simulink library "DQN_Lib"  (R2023b)
settings: Solver=VariableStepAuto  StartTime=0.0  StopTime=10.0  RelTol=1e-3
undefined symbols (not defined in the file): ACDC3, HRM, La, N, R, Ra, sps_AC, SYS, Ts, Ts_dqn, Ts_Power, w, Ws
libraries: DQN_Lib_bak x7
(part 3 of 3)

== matlab function DQN_Lib/Int_DQN/Int_d_2N_2 ==
  settings: updateMethod=DISCRETE
  data: Zdp output; Xdp input; Xdn input; Xdz input; Xqp input; Xqn input; Xqz input; Zdn output; N parameter; dt parameter; w parameter; EMT parameter; Zdz output; Zqp output; Zqn output; Zqz output; InitInt parameter; chkHrmLst parameter; HrmLst parameter
function [Zdp,Zdn,Zdz,Zqp,Zqn,Zqz]  = IntDQN(Xdp, Xdn, Xdz, Xqp, Xqn, Xqz, N, dt, w, EMT, InitInt, chkHrmLst, HrmLst)

    persistent Zdc_old;    
    persistent Xdc_old;   
    persistent Zdp_old;    
    persistent Zqp_old;    
    persistent Zdn_old;    
    persistent Zqn_old;    
    persistent Zdz_old;    
    persistent Zqz_old;  
       
    persistent HrmLst2;
    persistent dt2;
    persistent range;
    
    Xdc = zeros(6,1);
    Zdc = zeros(6,1);
    
    Xdc(1) = Xdp(1);
    Xdc(2) = Xdn(1);
    Xdc(3) = Xdz(1);
    Xdc(4) = Xqp(1);
    Xdc(5) = Xqn(1);
    Xdc(6) = Xqz(1);

    Xdp = [Xdp(2:end); zeros(N-numel(Xdp)+1,1)];
    Xqp = [Xqp(2:end); zeros(N-numel(Xqp)+1,1)];
    Xdn = [Xdn(2:end); zeros(N-numel(Xdn)+1,1)];
    Xqn = [Xqn(2:end); zeros(N-numel(Xqn)+1,1)];
    Xdz = [Xdz(2:end); zeros(N-numel(Xdz)+1,1)];
    Xqz = [Xqz(2:end); zeros(N-numel(Xqz)+1,1)];
       
    Zdp = zeros(N+1,1);
    Zdn = zeros(N+1,1);
    Zqp = zeros(N+1,1);
    Zqn = zeros(N+1,1);
    Zdz = zeros(N+1,1);
    Zqz = zeros(N+1,1);
    
    if(isempty(Zdc_old)) 
        Zdc_old  = InitInt';
        Xdc_old  = zeros(6,1);
        
        Zdp_old  = zeros(N,1); Zdp_old(1) = InitInt(1);
        Zdn_old  = zeros(N,1); Zdn_old(1) = InitInt(2);
        Zdz_old  = zeros(N,1); Zdz_old(1) = InitInt(3);
        Zqp_old  = zeros(N,1); Zqp_old(1) = InitInt(4);
        Zqn_old  = zeros(N,1); Zqn_old(1) = InitInt(5);
        Zqz_old  = zeros(N,1); Zqz_old(1) = InitInt(6);
        
        if(isempty(HrmLst2))            
            HrmLst2 = HrmLst;
            HrmLst2(HrmLst2==0) = [];
        end
        dt2 = dt/2;  
        
        if(chkHrmLst)
            range = numel(HrmLst2);
        else
            range = N; 
        end
        
    end

    
    
    Zdc(:) = dt2*(Xdc(:)+Xdc_old(:))+Zdc_old(:);
    Zdc_old = Zdc;
    Xdc_old = Xdc;


    if(N>0)
        A = 0;
        

        
        i = 1;

        for g = 1 : range
            
            if(chkHrmLst)
                if(HrmLst2(g)>0)
                    i = HrmLst2(g);
                end
            else
                i = g; 
            end
            
            
            wn =  i * w; 

            if(EMT)

                A = 2/(1+(dt2*wn)^2);
                %A = 1/(1+(dt2*wn)^2);

                wndt2 = wn*dt2;

                %%% POS %%%
                K1 = dt2*(2*Xdp(i)+Zqp_old(i)*wn) + Zdp_old(i);
                K2 = dt2*(2*Xqp(i)-Zdp_old(i)*wn) + Zqp_old(i);

                Zdp(i) = A*( K1 + wndt2*K2)/2;
                Zqp(i) = A*( K2 - wndt2*K1)/2;
                %Zdp(i) = A*( K1 + wndt2*K2);
                %Zqp(i) = A*( K2 - wndt2*K1);

                Zdp_old(i) = Zdp(i);
                Zqp_old(i) = Zqp(i); 

                %%% NEG %%%
                K1 = dt2*(2*Xdn(i)-Zqn_old(i)*wn) + Zdn_old(i);
                K2 = dt2*(2*Xqn(i)+Zdn_old(i)*wn) + Zqn_old(i);

                Zdn(i) = A*( K1 - wndt2*K2)/2;
                Zqn(i) = A*( K2 + wndt2*K1)/2;
                %Zdn(i) = A*( K1 - wndt2*K2);
                %Zqn(i) = A*( K2 + wndt2*K1);

                Zdn_old(i) = Zdn(i);
                Zqn_old(i) = Zqn(i);

                %%% ZERO %%%
                K1 = dt2*(2*Xdz(i)+Zqz_old(i)*wn) + Zdz_old(i);
                K2 = dt2*(2*Xqz(i)-Zdz_old(i)*wn) + Zqz_old(i);

                Zdz(i) = A*( K1 + wndt2*K2)/2;
                Zqz(i) = A*( K2 - wndt2*K1)/2;
                %Zdz(i) = A*( K1 + wndt2*K2);
                %Zqz(i) = A*( K2 - wndt2*K1);

                Zdz_old(i) = Zdz(i);
                Zqz_old(i) = Zqz(i);

            else
    
                Tad_p2 = (2/3)*[sin(0) sin(0-2*pi/3) sin(0+2*pi/3);  
                               cos(0) cos(0-2*pi/3) cos(0+2*pi/3);];

                Tad_z2 = (1/3)*[sin(0) sin(0) sin(0);  
                               cos(0) cos(0) cos(0);];

                Ta_dqn = [Tad_p2(1,:); Tad_p2(1,:); Tad_z2(1,:); Tad_p2(2,:); Tad_p2(2,:); Tad_z2(2,:)];

                Zdp(i) = (Xqp(i))*(1/(wn));
                Zqp(i) = (Xdp(i))*(-1/(wn)); 

                Zdn(i) = (Xqn(i))*(-1/(wn));
                Zqn(i) = (Xdn(i))*(1/(wn)); 

                Zdz(i) = (Xqz(i))*(1/(wn));
                Zqz(i) = (Xdz(i))*(-1/(wn));
                

                sT = sin(2*pi/3);
                cT = cos(2*pi/3);
%                 Zdc([1,4, 3]) = Zdc([1,4, 3])-Tad_p*[Zqp(i);-sT*Zdp(i)+cT*Zqp(i);sT*Zdp(i)+cT*Zqp(i)];
%                 Zdc([1,4, 3]) = Zdc([1,4, 3])-Tad_p*[Zqn(i);-sT*Zdn(i)+cT*Zqn(i);sT*Zdn(i)+cT*Zqn(i)];
%                 Zdc([1,4, 3]) = Zdc([1,4, 3])-Tad_p*[Zqz(i); Zqz(i)             ;Zqz(i)];

                Zdc = Zdc-Ta_dqn*[Zqp(i);-sT*Zdp(i)+cT*Zqp(i);sT*Zdp(i)+cT*Zqp(i)];
                Zdc = Zdc-Ta_dqn*[Zqn(i);-sT*Zdn(i)+cT*Zqn(i);sT*Zdn(i)+cT*Zqn(i)];
                Zdc = Zdc-Ta_dqn*[Zqz(i); Zqz(i)             ;Zqz(i)];

            end
            

        end

        Zdp(2:end) = Zdp(1:end-1);
        Zdn(2:end) = Zdn(1:end-1);
        Zdz(2:end) = Zdz(1:end-1);
        Zqp(2:end) = Zqp(1:end-1);
        Zqn(2:end) = Zqn(1:end-1);
        Zqz(2:end) = Zqz(1:end-1);


    end
    
    Zdp(1)     = Zdc(1);
    Zdn(1)     = Zdc(2);
    Zdz(1)     = Zdc(3);
    Zqp(1)     = Zdc(4);
    Zqn(1)     = Zdc(5);
    Zqz(1)     = Zdc(6);
end

== matlab function DQN_Lib/MATLAB Function9 ==
  data: Xdcpnz_c input; Y_DQN output
function Y_DQN  = f012C2DQN(Xdcpnz_c)

    if(size(Xdcpnz_c,2) < 2)
        error('Wrong size!');
    end
    
    N = size(Xdcpnz_c,2)-1;
    Y_DQN = zeros(N+1,6);

    Y_DQN(1,4) =  2*real(Xdcpnz_c(1,1));
    Y_DQN(1,5) =  2*real(Xdcpnz_c(2,1));
    Y_DQN(1,6) =  real(Xdcpnz_c(3,1));

    Y_DQN(1,1) =  -2*imag(Xdcpnz_c(1,1));
    Y_DQN(1,2) =  2*imag(Xdcpnz_c(2,1));
    Y_DQN(1,3) =  imag(Xdcpnz_c(3,1));
    
    for i = 2 : N + 1
    
        Y_DQN(i,1) =  real(Xdcpnz_c(1,i));
        Y_DQN(i,2) = -real(Xdcpnz_c(2,i));
        Y_DQN(i,3) =  real(Xdcpnz_c(3,i));

        Y_DQN(i,4) =  imag(Xdcpnz_c(1,i));
        Y_DQN(i,5) =  imag(Xdcpnz_c(2,i));
        Y_DQN(i,6) =  imag(Xdcpnz_c(3,i));
    
    end


end

== matlab function DQN_Lib/DQN2abc/DQn->ABC19 ==
  data: Xdp input; Xdn input; Xdz input; Xqp input; Xqn input; Xqz input; th input; abc output; N parameter
%function abc = Mult(Z0,Zdp,Zqp,Zdn,Zqn,Zdz,Zqz,th, N)
function abc = dqn2abc(Xdp,Xdn,Xdz,Xqp,Xqn,Xqz,th,N)

    %Xdc = zeros(1,6);
    Xdc = zeros(6,1);

    persistent Tda_p2;
    persistent Tdqn_a;
    
    if(isempty(Tda_p2)) 
        Tda_p2 = [-0           1     1;
                 -sqrt(3/4)  -0.5   1;
                  sqrt(3/4)  -0.5   1;];
                Tdqn_a = zeros(3,6);
                Tdqn_a = [Tda_p2(:,1)  Tda_p2(:,1)  0*Tda_p2(:,3)  Tda_p2(:,2)  Tda_p2(:,2)  2*Tda_p2(:,3)]/2;
    end


    Xdc(1) = Xdp(1);
    Xdc(2) = Xdn(1);
    Xdc(3) = Xdz(1);
    Xdc(4) = Xqp(1);
    Xdc(5) = Xqn(1);
    Xdc(6) = Xqz(1);

    abc = Tdqn_a*Xdc;

    abc3p = [0;0;0];
    abc3n = [0;0;0];
    abc1p = [0;0;0];
 

    for i = 1 : N

        Tda_p = [sin(i*th)          cos(i*th);
                 sin(i*th-2*pi/3)   cos(i*th-2*pi/3);
                 sin(i*th+2*pi/3)   cos(i*th+2*pi/3)];
        Tda_n = [sin(-i*th)         cos(-i*th);
                 sin(-i*th-2*pi/3)  cos(-i*th-2*pi/3);
                 sin(-i*th+2*pi/3)  cos(-i*th+2*pi/3)];
        Tda_z = [sin(i*th)          cos(i*th);
                 sin(i*th-0*pi/3)   cos(i*th-0*pi/3);
                 sin(i*th+0*pi/3)   cos(i*th+0*pi/3)];

        abc3p = abc3p + Tda_p*[Xdp(i+1);Xqp(i+1)];
        abc3n = abc3n + Tda_n*[Xdn(i+1);Xqn(i+1)];
        abc1p = abc1p + Tda_z*[Xdz(i+1);Xqz(i+1)];  

    end

    abc = abc+abc3p+abc3n+abc1p;%+abc1n;

== matlab function DQN_Lib/Add_DQN/MATLAB Function1 ==
  data: Xdp input; Xdn input; Xdz input; Xqp input; Xqn input; Xqz input; Ydp input; Ydn input; Ydz input; Yqp input; Yqn input; Yqz input; Zdp output; Zdn output; Zdz output; Zqp output; Zqn output; Zqz output; N parameter; chkHrmLst parameter; HrmLst parameter
function [Zdp,Zdn,Zdz,Zqp,Zqn,Zqz]  = SumDQN(Xdp, Xdn, Xdz, Xqp, Xqn, Xqz, Ydp, Ydn, Ydz, Yqp, Yqn, Yqz, N, chkHrmLst, HrmLst)
%function [Zdc,Zdp,Zqp,Zdn,Zqn,Zdz,Zqz]  = SumDQN(Xdc, Xdp, Xdn, Xdz, Xqp, Xqn, Xqz, Ydc, Ydp, Ydn, Ydz, Yqp, Yqn, Yqz, N)

    Xdp = [Xdp(1:end); zeros(N+1-numel(Xdp),1)];
    Ydp = [Ydp(1:end); zeros(N+1-numel(Ydp),1)];
    Xqp = [Xqp(1:end); zeros(N+1-numel(Xqp),1)];
    Yqp = [Yqp(1:end); zeros(N+1-numel(Yqp),1)];
      
    Xdn = [Xdn(1:end); zeros(N+1-numel(Xdn),1)];
    Ydn = [Ydn(1:end); zeros(N+1-numel(Ydn),1)];
    Xqn = [Xqn(1:end); zeros(N+1-numel(Xqn),1)];
    Yqn = [Yqn(1:end); zeros(N+1-numel(Yqn),1)];
    
    Xdz = [Xdz(1:end); zeros(N+1-numel(Xdz),1)];
    Ydz = [Ydz(1:end); zeros(N+1-numel(Ydz),1)];
    Xqz = [Xqz(1:end); zeros(N+1-numel(Xqz),1)];
    Yqz = [Yqz(1:end); zeros(N+1-numel(Yqz),1)];
       
    Zdp = zeros(N+1,1);
    Zdn = zeros(N+1,1);
    Zqp = zeros(N+1,1);
    Zqn = zeros(N+1,1);
    Zdz = zeros(N+1,1);
    Zqz = zeros(N+1,1);
    
    persistent range;
    
    if(isempty(range))        
        if(chkHrmLst)
            range = numel(HrmLst);
        else
            range = N+1; 
        end
    end
         
    h = 1;
    
    for i = 1 : range
        
        if(chkHrmLst)
            if(HrmLst(i)>0)
                h = HrmLst(i)+1;
            end
        else
            h = i; 
        end
        
        Zdp(h) = Xdp(h)+Ydp(h);
        Zdn(h) = Xdn(h)+Ydn(h);
        Zqp(h) = Xqp(h)+Yqp(h);
        Zqn(h) = Xqn(h)+Yqn(h);
        Zdz(h) = Xdz(h)+Ydz(h);
        Zqz(h) = Xqz(h)+Yqz(h);
    end
end

== matlab function DQN_Lib/MATLAB Function1 ==
  data: u input; y output size=33 [1..100]; Ad parameter; Bd parameter; Cd parameter; Dd parameter; dt parameter; nsw parameter; InitVec parameter; bvec input
function y = DSS(u, Ad, Bd, Cd, Dd, dt, nsw, InitVec, bvec)

% INIT
x = zeros(size(Ad,1),1);
y = zeros(size(Cd,1),1);
%bvec_old = zeros(2,1);

persistent Ad11;
persistent Ad12;
persistent Ad21;
persistent Ad22;

persistent Bd11;
persistent Bd12;
persistent Bd21;
persistent Bd22;
persistent Cd11;
persistent Cd12;
persistent Cd21;
persistent Cd22;
persistent Dd11;
persistent Dd12;
persistent Dd21;
persistent Dd22;

persistent Ads;
persistent Bds;
persistent Cds;
persistent Dds;

persistent x_old;
persistent bvec_old;

persistent nrSt;
persistent nrOut;

    
    if(isempty(x_old))

        nrSt = size(Ad,1);
        nrOut = size(Cd,1);

        % swFlag = 0;
        % 
        % arows = size(Ad,1)/3; %signal size
        % acols = size(Ad,2)/3; %signal size
        % 
        % brows = size(Bd,1)/3; %signal size
        % bcols = size(Bd,2)/3; %signal size
        % 
        % crows = size(Cd,1)/3; %signal size
        % ccols = size(Cd,2)/3; %signal size
        % 
        % drows = size(Dd,1)/3; %signal size
        % dcols = size(Dd,2)/3; %signal size
        
        Ad11 = Ad(1:nsw,1:nsw);        if(isempty(Ad11)) Ad11 = zeros(3,3); end
        Ad12 = Ad(1:nsw,nsw+1:end);    if(isempty(Ad12)) Ad12 = zeros(3,3); end
        Ad21 = Ad(nsw+1:end,1:nsw);    if(isempty(Ad21)) Ad21 = zeros(3,3); end
        Ad22 = Ad(nsw+1:end,nsw+1:end); if(isempty(Ad22)) Ad22 = zeros(3,3); end
        
        Bd11 = Bd(1:nsw,1:nsw);        if(isempty(Bd11)) Bd11 = zeros(3,3); end
        Bd12 = Bd(1:nsw,nsw+1:end);    if(isempty(Bd12)) Bd12 = zeros(3,3); end
        Bd21 = Bd(nsw+1:end,1:nsw);    if(isempty(Bd21)) Bd21 = zeros(3,3); end
        Bd22 = Bd(nsw+1:end,nsw+1:end); if(isempty(Bd22)) Bd22 = zeros(3,size(Bd,2)-nsw); end
        
        Cd11 = Cd(1:nsw,1:nsw);        if(isempty(Cd11)) Cd11 = zeros(3,3); end
        Cd12 = Cd(1:nsw,nsw+1:end);    if(isempty(Cd12)) Cd12 = zeros(3,3); end
        Cd21 = Cd(nsw+1:end,1:nsw);    if(isempty(Cd21)) Cd21 = zeros(3,3); end
        Cd22 = Cd(nsw+1:end,nsw+1:end); if(isempty(Cd22)) Cd22 = zeros(size(Cd,1)-nsw,size(Cd,2)); end
        
        Dd11 = Dd(1:nsw,1:nsw);        if(isempty(Dd11)) Dd11 = zeros(3,3); end
        Dd12 = Dd(1:nsw,nsw+1:end);    if(isempty(Dd12)) Dd12 = zeros(3,3); end
        Dd21 = Dd(nsw+1:end,1:nsw);    if(isempty(Dd21)) Dd21 = zeros(3,3); end
        Dd22 = Dd(nsw+1:end,nsw+1:end); if(isempty(Dd22)) Dd22 = zeros(3,3); end
        
        x_old = zeros(size(Ad,1),1);
        bvec_old = bvec;     

        kb1 = 1e6*abs(1-bvec(1))+0.01*abs(0-bvec(1));
        kb2 = 1e6*abs(1-bvec(2))+0.01*abs(0-bvec(2));

        Dd11k = [Dd11(:,1:3)/kb1 Dd11(:,4:6)/kb2];
        D11Ik = eye(nsw)/(eye(nsw) - Dd11k);
        Dd21k = [Dd21(:,1:3)/kb1 Dd21(:,4:6)/kb2];
        
        E = D11Ik * Cd11;
        F = D11Ik * Cd12;
        I = D11Ik*Dd12;
      
        
        Bd11k = [Bd11(:,1:3)/kb1 Bd11(:,4:6)/kb2];
        Bd21k = [Bd21(:,1:3)/kb1 Bd21(:,4:6)/kb2];

        Ads = [Ad11+Bd11k*E Ad12+Bd11k*F ; Ad21+Bd21k*E Ad22+Bd21k*F ];
        Bds = [(Bd11k*I + Bd12); Bd21k*I + Bd22];
        Cds = [ D11Ik * Cd11 D11Ik * Cd12 ; Dd21k*D11Ik*Cd11 + Cd21 Dd21k*D11Ik*Cd12 + Cd22];
        Dds = [ D11Ik*Dd12; (Dd22+Dd21k*D11Ik*Dd12)];
    
    end


    if(any(bvec_old ~= bvec))
        kb1 = 1e6*abs(1-bvec(1))+0.01*abs(0-bvec(1));
        kb2 = 1e6*abs(1-bvec(2))+0.01*abs(0-bvec(2));

        Dd11k = [Dd11(:,1:3)/kb1 Dd11(:,4:6)/kb2];
        D11Ik = eye(nsw)/(eye(nsw) - Dd11k);
        Dd21k = [Dd21(:,1:3)/kb1 Dd21(:,4:6)/kb2];
        
        E = D11Ik * Cd11;
        F = D11Ik * Cd12;
        I = D11Ik*Dd12;
      
        
        Bd11k = [Bd11(:,1:3)/kb1 Bd11(:,4:6)/kb2];
        Bd21k = [Bd21(:,1:3)/kb1 Bd21(:,4:6)/kb2];

        Ads = [Ad11+Bd11k*E Ad12+Bd11k*F ; Ad21+Bd21k*E Ad22+Bd21k*F ];
        Bds = [(Bd11k*I + Bd12); Bd21k*I + Bd22];
        Cds = [ D11Ik * Cd11 D11Ik * Cd12 ; Dd21k*D11Ik*Cd11 + Cd21 Dd21k*D11Ik*Cd12 + Cd22];
        Dds = [ D11Ik*Dd12; (Dd22+Dd21k*D11Ik*Dd12)];
    end


    x = Ads*x_old   + Bds*u(nsw+1:end);                                                     
    y(1:nrOut) = Cds*x       + Dds*u(nsw+1:end);        



    %OLD
    x_old(1:nrSt) = x(1:nrSt);
    bvec_old(1:2) = bvec(1:2);





end
